simulink model "SingleStreamSSRwithPL"  (R2021a)
settings: Solver=VariableStepAuto  StartTime=0.0  StopTime=inf  RelTol=1e-3
PreLoadFcn:
  | xmcCheckSlxPath(bdroot)
  | SSR4_init
InitFcn:
  | xmcCheckSlxPath(bdroot)
  | SSR4_init;
undefined symbols (not defined in the file): c, FIR_MultiKernel_cin, FIR_MultiKernel_cincout, FIR_MultiKernel_cout, FramesPerVector, S, SHIFT_ACC, SingleStream, T, Taps, ValidDelay, VectorSize, vsva2197, xcvc1902
libraries: hdlBasic x84, aieBasic x28, simulink x25, aieUtilities x12, dspsrcs4 x1, vmcUtilities x1
(part 1 of 3)
settings Model: Creator=oliviert  LastModifiedBy=abehbood
settings SolverCC: AlgebraicLoopSolver=TrustRegion
settings DebuggingCC: SFMachineParentedDataDiag=warning

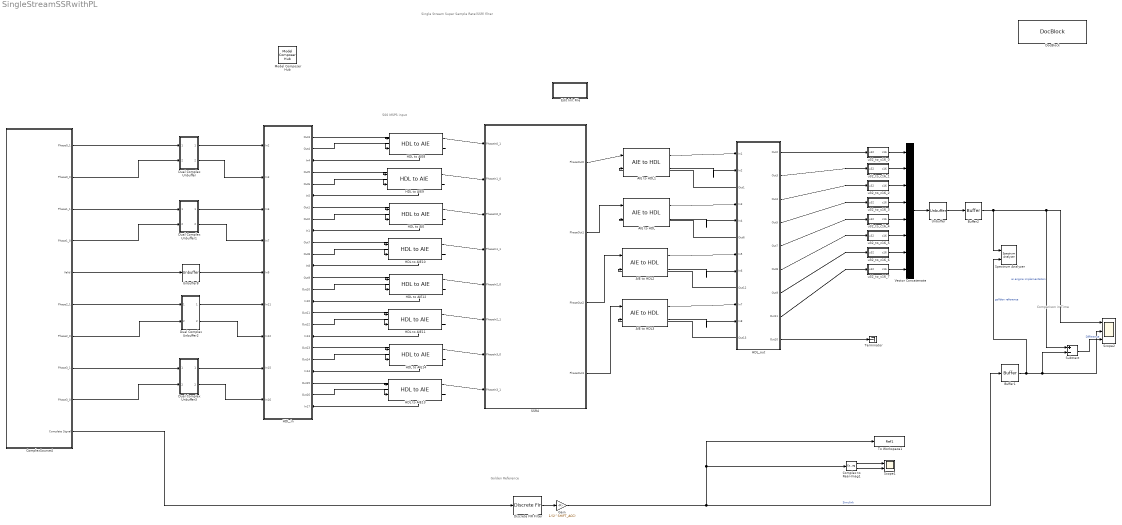
== system SingleStreamSSRwithPL ==
  note: Golden Reference
  note: Single Stream Super Sample Rate(SSR) filter
  note: Comparison in Time
  note: 500 MSPS input
  AIE to HDL{,1..3} (4 alike) : aieUtilities/AIE to HDL  OutDataType=uint64  OutSampleTime=1
  Buffer1 : Buffer  N=16  OutputFrames=off
  Buffer2 : Buffer  N=16  OutputFrames=off
  Complex to Real-Imag1 : ComplexToRealImag
  ComplexSource4 : Subsystem  mask{s=0}
      mask prompts: s "Seed"
  Discrete FIR Filter : DiscreteFir  Coefficients=Taps  InputProcessing=Columns as channels (frame based)
  DocBlock : simulink/Model-Wide Utilities/DocBlock  DocumentType=Text  mask(DocBlock){}
      content=|
      | ///////////////////////////////////////////////////////////////////////////
      | // Copyright 2020 Xilinx
      | //
      | // Licensed under the Apache License, Version 2.0 (the "License");
      | // you may not use this file except in compliance with the License.
      | // You may obtain a copy of the License at
      | //
      | // http://www.apache.org/licenses/LICENSE-2.0
      | //
      | // Unless required by applicable law or agreed to in writing, software
      | // distributed under the License is distributed on an "AS IS" BASIS,
      | // WITHOUT WARRANTIES OR CONDITIONS OF ANY KIND, either express or implied.
      | // See the License for the specific language governing permissions and
      | // limitations under the License.
      | ///////////////////////////////////////////////////////////////////////////
      mask Display:
      | xmcDrawBlockIcon();
      | disp(['{\fontsize{10pt}(c) Copyright 2020' ' Xilinx, Inc.}\newline \newline '],'texmode','on');
      | disp('{\fontsize{10pt}Licensed under the Apache License 2.0}','texmode','on');
      | disp('\newline \newline \newline{\fontsize{10pt}Double Click for Copyright Notice}','texmode','on');
  Dual Complex Unbuffer : Subsystem
  Dual Complex Unbuffer1 : Subsystem
  Dual Complex Unbuffer2 : Subsystem
  Dual Complex Unbuffer3 : Subsystem
  Edit Init File : Subsystem
      settings: OpenFcn=edit('SSR4_init.m');
  Gain : Gain  Gain=1/(2^SHIFT_ACC)
  HDL to AIE{,8..14} (8 alike) : aieUtilities/HDL to AIE  OutDataType=int16 (c)  OutSampleTime=4/T  SamplesPerFrame=4
  HDL_in : Subsystem
      settings: PortSchema="{\"entries\":[{\"content\":{\"sides\":[{\"content\":{\"connectorIds\":[\"In1\",\"In2\",\"In3\",\"In4\",\"In5\",\"In6\",\"In7\",\"In8\",\"In9\"]},\"type\":\"ConnectorPlacement.EquallySpacedRectSide\",\"uuid\":\"43963710-6fd6-4ca2-aef5-f578b9dcb653\"},{\"content\":{\"connectorIds\":[\"Out1\",\"Out2\",\"In10\",\"Out3\",\"Out4\",\"In11\",\"Out5\",\"Out6\",\"In12\",\"Out7\",\"Out8\",\"In13\",\"Out9\",\"Out10\",\"In14\",\"Out11\",\"Out12\",\"In15\",\"Out13\",\"Out14\",\"In16\",\"Out15\",\"Out16\",\"In17\"],\"side\":\"RIGHT\"},\"type\":\"ConnectorPlacement.EquallySpacedRectSide\",\"uuid\":\"a4fb1d0d-700c-40f1-8501-f280c21d0c52\"},{\"content\":{\"connectorIds\":[],\"side\":\"TOP\"},\"type\":\"ConnectorPlacement.EquallySpacedRectSide\",\"uuid\":\"ff581830-d8dd-44d7-ae40-7c0c1ac080ec\"}]},\"type\":\"ConnectorPlacement.EquallySpacedConnector\",\"uuid\":\"e2183898-06e4-482e-ae06-3d392b216275\"}],\"packageUris\":[\"http://schema.mathworks.com/mf0/Connector/R2020b\"],\"version\":\"1.0\"}"
  HDL_out : Subsystem
      settings: PortSchema="{\"entries\":[{\"content\":{\"sides\":[{\"content\":{\"connectorIds\":[\"In1\",\"In2\",\"Out10\",\"In3\",\"In4\",\"Out11\",\"In5\",\"In6\",\"Out12\",\"In7\",\"In8\",\"Out13\"]},\"type\":\"ConnectorPlacement.EquallySpacedRectSide\",\"uuid\":\"7f2474ee-a2a5-4d74-ae03-57eff4eca528\"},{\"content\":{\"connectorIds\":[\"Out1\",\"Out2\",\"Out3\",\"Out4\",\"Out5\",\"Out6\",\"Out7\",\"Out8\",\"Out9\"],\"side\":\"RIGHT\"},\"type\":\"ConnectorPlacement.EquallySpacedRectSide\",\"uuid\":\"05904fba-80d7-4be6-91c3-65cee4e3c770\"},{\"content\":{\"connectorIds\":[],\"side\":\"TOP\"},\"type\":\"ConnectorPlacement.EquallySpacedRectSide\",\"uuid\":\"ee8e52c5-3092-4f59-816b-8523dabda97a\"}]},\"type\":\"ConnectorPlacement.EquallySpacedConnector\",\"uuid\":\"7b2a5572-57fc-4b8c-a1f0-10ceb4480a97\"}],\"packageUris\":[\"http://schema.mathworks.com/mf0/Connector/R2020b\"],\"version\":\"1.0\"}"
  Model Composer Hub : vmcUtilities/Model Composer Hub  Tag=genX  CodeGeneration=off  SubsystemName=SSR4  TargetDirectory=./code  ExportType=AI Engines  IpVendor=xilinx.com  IpLibrary=hls  IpVersion=1.0  IpHWLanguage=Verilog  AieCompilerOptions={}  CreateTestbench=off  TestbenchStackSize=10  RunAieSim=off  AieSimTimeout=50000  RunAieSimProfiling=off  LaunchVitisAnalyzer=off  PlotOutput=off  RunX86Sim=off  X86SimTimeout=10  GenHwImage=off  PlatformType=Specify Platform  Platform=/proj/xbuilds/SWIP/2022.1_0310_2135/installs/lin64/Vitis/2022.1/base_platforms/xilinx_vck190_base_202210_1/xilinx_vck190_base_202210_1.xpfm  HwSystemType=Baremetal  HwValidationTarget=hw  ProjDevice=Versal VCK190 Evaluation Platform (xcvc1902-vsva2197-2MP-e-S)  ProjDevicePart=xcvc1902-vsva2197-2MP-e-S  SamplePeriod=-1  ClockFrequency=200  DataPathParallelism=1  xilinxfamily=versalaicore  part=xcvc1902  speed=-2MP-e-S  package=vsva2197  directory=./netlist  testbench=off  incr_netlist=off  synthesis_tool=Vivado  clock_wrapper=Clock Enables  dbl_ovrd=According to Block Masks  dcm_input_clock_period=10  sysclk_period=10  simulink_period=1  eval_field=0
  SSR4 : Subsystem
  Scope1 : Scope  NumInputPorts=2
  Scope2 : Scope  NumInputPorts=3
  Spectrum Analyzer : SpectrumAnalyzer  NumInputPorts=2
  Subtract : Sum  Inputs=+-
  Terminator : Terminator
  To Workspace1 : ToWorkspace  VariableName=Ref1  SampleTime=-1
      settings: Save2DSignal=2-D array (concatenate along first dimension)
  Unbuffer : Unbuffer
  Unbuffer8 : Unbuffer
  Vector Concatenate : Concatenate  NumInputs=8
  u32_to_c16_0 : Subsystem
  u32_to_c16_1 : Subsystem
  u32_to_c16_2 : Subsystem
  u32_to_c16_3 : Subsystem
  u32_to_c16_4 : Subsystem
  u32_to_c16_5 : Subsystem
  u32_to_c16_6 : Subsystem
  u32_to_c16_7 : Subsystem
  wires:
  ComplexSource4/10(Complete Signal) -> Discrete FIR Filter/1
  Discrete FIR Filter/1 -> Gain/1
  HDL to AIE/1 -> SSR4/3(PhaseIn0_0)
  HDL to AIE8/1 -> SSR4/1(PhaseIn0_1)
  HDL to AIE9/1 -> SSR4/2(PhaseIn1_0)
  HDL to AIE10/1 -> SSR4/4(PhaseIn1_1)
  HDL to AIE12/1 -> SSR4/5(PhaseIn2_0)
  HDL to AIE11/1 -> SSR4/6(PhaseIn2_1)
  HDL to AIE14/1 -> SSR4/7(PhaseIn3_0)
  HDL to AIE13/1 -> SSR4/8(PhaseIn3_1)
  Subtract/1 -> Scope2/3  "Difference"
  Complex to Real-Imag1/2 -> Scope1/2
  Complex to Real-Imag1/1 -> Scope1/1
  Gain/1 -> To Workspace1/1, Complex to Real-Imag1/1, Buffer1/1  "Simulink"
  Buffer1/1 -> Subtract/2, Scope2/2, Spectrum Analyzer/2  "gollden reference"
  Unbuffer/1 -> Buffer2/1
  Buffer2/1 -> Subtract/1, Scope2/1, Spectrum Analyzer/1  "ai engine implementation"
  ComplexSource4/1(Phase0_1) -> Dual Complex Unbuffer/1(P0_1)
  ComplexSource4/9(Phase3_0) -> Dual Complex Unbuffer3/2(P0_0)
  ComplexSource4/8(Phase3_1) -> Dual Complex Unbuffer3/1(P0_1)
  ComplexSource4/7(Phase2_0) -> Dual Complex Unbuffer2/2(P0_0)
  ComplexSource4/6(Phase2_1) -> Dual Complex Unbuffer2/1(P0_1)
  ComplexSource4/4(Phase1_0) -> Dual Complex Unbuffer1/2(P0_0)
  ComplexSource4/3(Phase1_1) -> Dual Complex Unbuffer1/1(P0_1)
  ComplexSource4/5(Valid) -> Unbuffer8/1
  ComplexSource4/2(Phase0_0) -> Dual Complex Unbuffer/2(P0_0)
  HDL to AIE/2 -> HDL_in/12(In1)
  Dual Complex Unbuffer/1(Out1) -> HDL_in/1(In2)
  Dual Complex Unbuffer/2(Out2) -> HDL_in/2(In3)
  HDL to AIE8/2 -> HDL_in/10(In4)
  HDL to AIE9/2 -> HDL_in/11(In5)
  Dual Complex Unbuffer1/1(Out1) -> HDL_in/3(In6)
  Dual Complex Unbuffer1/2(Out2) -> HDL_in/4(In7)
  HDL to AIE10/2 -> HDL_in/13(In8)
  Unbuffer8/1 -> HDL_in/5(In9)
  HDL to AIE12/2 -> HDL_in/14(In10)
  Dual Complex Unbuffer2/1(Out1) -> HDL_in/6(In11)
  Dual Complex Unbuffer2/2(Out2) -> HDL_in/7(In12)
  HDL to AIE11/2 -> HDL_in/15(In13)
  HDL to AIE14/2 -> HDL_in/16(In14)
  Dual Complex Unbuffer3/1(Out1) -> HDL_in/8(In15)
  Dual Complex Unbuffer3/2(Out2) -> HDL_in/9(In16)
  HDL to AIE13/2 -> HDL_in/17(In17)
  HDL_in/5(Out1) -> HDL to AIE/1
  HDL_in/6(Out2) -> HDL to AIE/2
  HDL_in/1(Out3) -> HDL to AIE8/1
  HDL_in/2(Out4) -> HDL to AIE8/2
  HDL_in/3(Out5) -> HDL to AIE9/1
  HDL_in/4(Out6) -> HDL to AIE9/2
  HDL_in/7(Out7) -> HDL to AIE10/1
  HDL_in/8(Out8) -> HDL to AIE10/2
  HDL_in/9(Out9) -> HDL to AIE12/1
  HDL_in/10(Out10) -> HDL to AIE12/2
  HDL_in/11(Out11) -> HDL to AIE11/1
  HDL_in/12(Out12) -> HDL to AIE11/2
  HDL_in/13(Out13) -> HDL to AIE14/1
  HDL_in/14(Out14) -> HDL to AIE14/2
  HDL_in/15(Out15) -> HDL to AIE13/1
  HDL_in/16(Out16) -> HDL to AIE13/2
  u32_to_c16_7/1(c16) -> Vector Concatenate/8
  u32_to_c16_6/1(c16) -> Vector Concatenate/7
  u32_to_c16_5/1(c16) -> Vector Concatenate/6
  u32_to_c16_4/1(c16) -> Vector Concatenate/5
  u32_to_c16_3/1(c16) -> Vector Concatenate/4
  u32_to_c16_2/1(c16) -> Vector Concatenate/3
  u32_to_c16_1/1(c16) -> Vector Concatenate/2
  u32_to_c16_0/1(c16) -> Vector Concatenate/1
  Vector Concatenate/1 -> Unbuffer/1
  SSR4/4(PhaseOut3) -> AIE to HDL3/1
  SSR4/3(PhaseOut2) -> AIE to HDL2/1
  SSR4/2(PhaseOut1) -> AIE to HDL/1
  SSR4/1(PhaseOut0) -> AIE to HDL1/1
  AIE to HDL1/1 -> HDL_out/1(In1)
  AIE to HDL1/2 -> HDL_out/2(In2)
  AIE to HDL/1 -> HDL_out/3(In3)
  AIE to HDL/2 -> HDL_out/4(In4)
  AIE to HDL2/1 -> HDL_out/5(In5)
  AIE to HDL2/2 -> HDL_out/6(In6)
  AIE to HDL3/1 -> HDL_out/7(In7)
  AIE to HDL3/2 -> HDL_out/8(In8)
  HDL_out/10(Out1) -> AIE to HDL1/2
  HDL_out/1(Out2) -> u32_to_c16_0/1(u32)
  HDL_out/2(Out3) -> u32_to_c16_1/1(u32)
  HDL_out/3(Out4) -> u32_to_c16_2/1(u32)
  HDL_out/4(Out5) -> u32_to_c16_3/1(u32)
  HDL_out/11(Out6) -> AIE to HDL/2
  HDL_out/5(Out7) -> u32_to_c16_4/1(u32)
  HDL_out/6(Out8) -> u32_to_c16_5/1(u32)
  HDL_out/7(Out9) -> u32_to_c16_6/1(u32)
  HDL_out/9(Out10) -> Terminator/1
  HDL_out/8(Out11) -> u32_to_c16_7/1(u32)
  HDL_out/12(Out12) -> AIE to HDL2/2
  HDL_out/13(Out13) -> AIE to HDL3/2

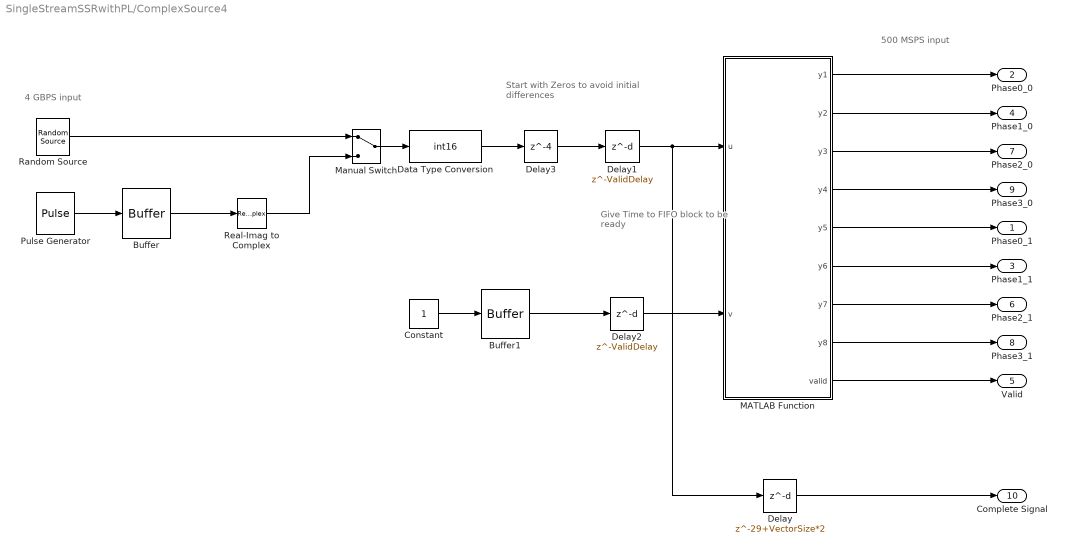
== system SingleStreamSSRwithPL/ComplexSource4 ==
  note: Give Time to
      | FIFO block
      | to be ready
  note: Start with Zeros
      | to avoid
      | initial differences
  note: 4 GBPS input
  note: 500 MSPS input
  Buffer : Buffer  N=VectorSize  OutputFrames=off
  Buffer1 : Buffer  N=FramesPerVector  OutputFrames=off
  Constant : Constant  SampleTime=1
  Data Type Conversion : DataTypeConversion  OutDataTypeStr=int16
  Delay : Delay  DelayLength=29+VectorSize*2  InputProcessing=Columns as channels (frame based)
  Delay1 : Delay  DelayLength=ValidDelay
  Delay2 : Delay  DelayLength=ValidDelay
  Delay3 : Delay  DelayLength=4
  MATLAB Function : MATLAB Function  TreatAsAtomicUnit=on
  Manual Switch : ManualSwitch
  Pulse Generator : DiscretePulseGenerator  Amplitude=20000  Period=32 + 40*5  PhaseDelay=32  SampleTime=1/T
  Random Source : dspsrcs4/Random Source  SrcType=Uniform  NormMethod=Ziggurat  CltLength=12  MinVal=-20000  MaxVal=20000  MeanVal=0  VarVal=1  RepMode=Specify seed  rawSeed=s  IsInherit=off  SampMode=Discrete  SampTime=1/T  SampFrame=VectorSize  DataType=Double  OutComplex=Complex  OutputFrames=off
  Real-Imag to Complex : RealImagToComplex  Input=Real
  Phase0_1 : Outport
  Phase0_0 : Outport  Port=2
  Phase1_1 : Outport  Port=3
  Phase1_0 : Outport  Port=4
  Valid : Outport  Port=5
  Phase2_1 : Outport  Port=6
  Phase2_0 : Outport  Port=7
  Phase3_1 : Outport  Port=8
  Phase3_0 : Outport  Port=9
  Complete Signal : Outport  Port=10
  wires:
  MATLAB Function/1(y1) -> Phase0_0/1
  MATLAB Function/2(y2) -> Phase1_0/1
  MATLAB Function/3(y3) -> Phase2_0/1
  MATLAB Function/4(y4) -> Phase3_0/1
  Real-Imag to Complex/1 -> Manual Switch/2
  Pulse Generator/1 -> Buffer/1
  Delay/1 -> Complete Signal/1
  Buffer/1 -> Real-Imag to Complex/1
  Manual Switch/1 -> Data Type Conversion/1
  MATLAB Function/9(valid) -> Valid/1
  MATLAB Function/8(y8) -> Phase3_1/1
  MATLAB Function/7(y7) -> Phase2_1/1
  MATLAB Function/6(y6) -> Phase1_1/1
  MATLAB Function/5(y5) -> Phase0_1/1
  Random Source/1 -> Manual Switch/1
  Delay1/1 -> Delay/1, MATLAB Function/1(u)
  Delay2/1 -> MATLAB Function/2(v)
  Constant/1 -> Buffer1/1
  Buffer1/1 -> Delay2/1
  Data Type Conversion/1 -> Delay3/1
  Delay3/1 -> Delay1/1

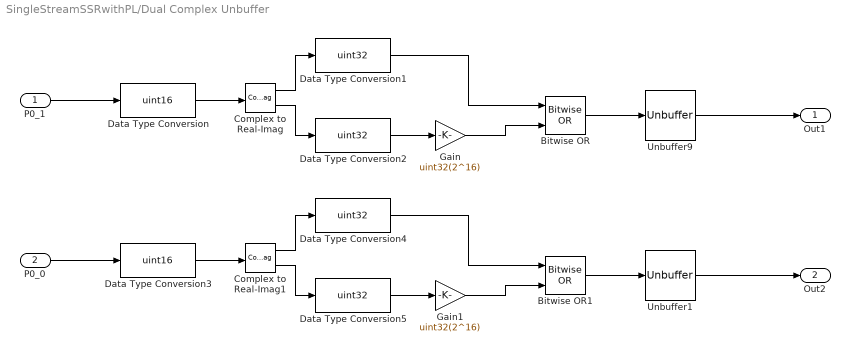
== system SingleStreamSSRwithPL/Dual Complex Unbuffer ==
  P0_1 : Inport
  P0_0 : Inport  Port=2
  Bitwise OR : simulink/Logic and Bit Operations/Bitwise Operator  logicop=OR  UseBitMask=off  NumInputPorts=2  BitMask=bin2dec('11011001')  BitMaskRealWorld=Stored Integer
  Bitwise OR1 : simulink/Logic and Bit Operations/Bitwise Operator  logicop=OR  UseBitMask=off  NumInputPorts=2  BitMask=bin2dec('11011001')  BitMaskRealWorld=Stored Integer
  Complex to Real-Imag : ComplexToRealImag
  Complex to Real-Imag1 : ComplexToRealImag
  Data Type Conversion : DataTypeConversion  OutDataTypeStr=uint16  ConvertRealWorld=Stored Integer (SI)
  Data Type Conversion{1..2,4..5} (4 alike) : DataTypeConversion  OutDataTypeStr=uint32  ConvertRealWorld=Stored Integer (SI)
  Data Type Conversion3 : DataTypeConversion  OutDataTypeStr=uint16  ConvertRealWorld=Stored Integer (SI)
  Gain : Gain  Gain=uint32(2^16)  OutDataTypeStr=uint32
  Gain1 : Gain  Gain=uint32(2^16)  OutDataTypeStr=uint32
  Unbuffer1 : Unbuffer
  Unbuffer9 : Unbuffer
  Out1 : Outport
  Out2 : Outport  Port=2
  wires:
  Unbuffer1/1 -> Out2/1
  Unbuffer9/1 -> Out1/1
  Data Type Conversion/1 -> Complex to Real-Imag/1
  P0_1/1 -> Data Type Conversion/1
  Data Type Conversion2/1 -> Gain/1
  Bitwise OR/1 -> Unbuffer9/1
  Complex to Real-Imag/1 -> Data Type Conversion1/1
  Complex to Real-Imag/2 -> Data Type Conversion2/1
  Data Type Conversion1/1 -> Bitwise OR/1
  Gain/1 -> Bitwise OR/2
  Gain1/1 -> Bitwise OR1/2
  Data Type Conversion4/1 -> Bitwise OR1/1
  Complex to Real-Imag1/2 -> Data Type Conversion5/1
  Complex to Real-Imag1/1 -> Data Type Conversion4/1
  Data Type Conversion5/1 -> Gain1/1
  Data Type Conversion3/1 -> Complex to Real-Imag1/1
  P0_0/1 -> Data Type Conversion3/1
  Bitwise OR1/1 -> Unbuffer1/1

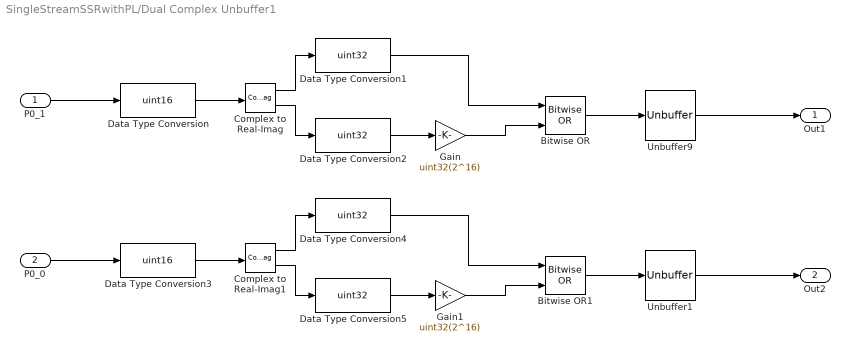
== system SingleStreamSSRwithPL/Dual Complex Unbuffer1 ==
  P0_1 : Inport
  P0_0 : Inport  Port=2
  Bitwise OR : simulink/Logic and Bit Operations/Bitwise Operator  logicop=OR  UseBitMask=off  NumInputPorts=2  BitMask=bin2dec('11011001')  BitMaskRealWorld=Stored Integer
  Bitwise OR1 : simulink/Logic and Bit Operations/Bitwise Operator  logicop=OR  UseBitMask=off  NumInputPorts=2  BitMask=bin2dec('11011001')  BitMaskRealWorld=Stored Integer
  Complex to Real-Imag : ComplexToRealImag
  Complex to Real-Imag1 : ComplexToRealImag
  Data Type Conversion : DataTypeConversion  OutDataTypeStr=uint16  ConvertRealWorld=Stored Integer (SI)
  Data Type Conversion{1..2,4..5} (4 alike) : DataTypeConversion  OutDataTypeStr=uint32  ConvertRealWorld=Stored Integer (SI)
  Data Type Conversion3 : DataTypeConversion  OutDataTypeStr=uint16  ConvertRealWorld=Stored Integer (SI)
  Gain : Gain  Gain=uint32(2^16)  OutDataTypeStr=uint32
  Gain1 : Gain  Gain=uint32(2^16)  OutDataTypeStr=uint32
  Unbuffer1 : Unbuffer
  Unbuffer9 : Unbuffer
  Out1 : Outport
  Out2 : Outport  Port=2
  wires:
  Bitwise OR1/1 -> Unbuffer1/1
  P0_0/1 -> Data Type Conversion3/1
  Data Type Conversion3/1 -> Complex to Real-Imag1/1
  Data Type Conversion5/1 -> Gain1/1
  Complex to Real-Imag1/1 -> Data Type Conversion4/1
  Complex to Real-Imag1/2 -> Data Type Conversion5/1
  Data Type Conversion4/1 -> Bitwise OR1/1
  Gain1/1 -> Bitwise OR1/2
  Gain/1 -> Bitwise OR/2
  Data Type Conversion1/1 -> Bitwise OR/1
  Complex to Real-Imag/2 -> Data Type Conversion2/1
  Complex to Real-Imag/1 -> Data Type Conversion1/1
  Bitwise OR/1 -> Unbuffer9/1
  Data Type Conversion2/1 -> Gain/1
  P0_1/1 -> Data Type Conversion/1
  Data Type Conversion/1 -> Complex to Real-Imag/1
  Unbuffer9/1 -> Out1/1
  Unbuffer1/1 -> Out2/1

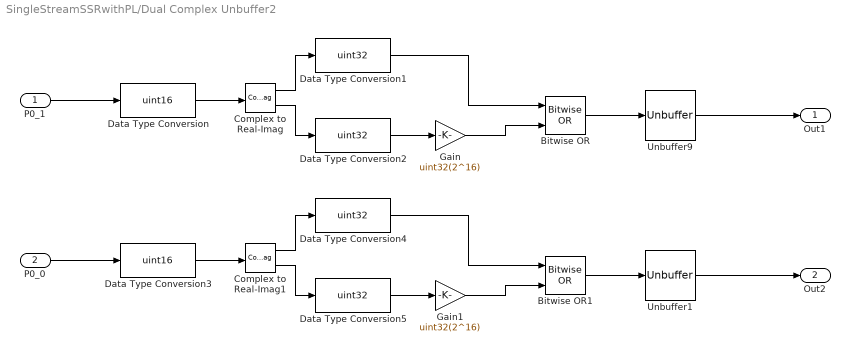
== system SingleStreamSSRwithPL/Dual Complex Unbuffer2 ==
  P0_1 : Inport
  P0_0 : Inport  Port=2
  Bitwise OR : simulink/Logic and Bit Operations/Bitwise Operator  logicop=OR  UseBitMask=off  NumInputPorts=2  BitMask=bin2dec('11011001')  BitMaskRealWorld=Stored Integer
  Bitwise OR1 : simulink/Logic and Bit Operations/Bitwise Operator  logicop=OR  UseBitMask=off  NumInputPorts=2  BitMask=bin2dec('11011001')  BitMaskRealWorld=Stored Integer
  Complex to Real-Imag : ComplexToRealImag
  Complex to Real-Imag1 : ComplexToRealImag
  Data Type Conversion : DataTypeConversion  OutDataTypeStr=uint16  ConvertRealWorld=Stored Integer (SI)
  Data Type Conversion{1..2,4..5} (4 alike) : DataTypeConversion  OutDataTypeStr=uint32  ConvertRealWorld=Stored Integer (SI)
  Data Type Conversion3 : DataTypeConversion  OutDataTypeStr=uint16  ConvertRealWorld=Stored Integer (SI)
  Gain : Gain  Gain=uint32(2^16)  OutDataTypeStr=uint32
  Gain1 : Gain  Gain=uint32(2^16)  OutDataTypeStr=uint32
  Unbuffer1 : Unbuffer
  Unbuffer9 : Unbuffer
  Out1 : Outport
  Out2 : Outport  Port=2
  wires:
  Bitwise OR1/1 -> Unbuffer1/1
  P0_0/1 -> Data Type Conversion3/1
  Data Type Conversion3/1 -> Complex to Real-Imag1/1
  Data Type Conversion5/1 -> Gain1/1
  Complex to Real-Imag1/1 -> Data Type Conversion4/1
  Complex to Real-Imag1/2 -> Data Type Conversion5/1
  Data Type Conversion4/1 -> Bitwise OR1/1
  Gain1/1 -> Bitwise OR1/2
  Gain/1 -> Bitwise OR/2
  Data Type Conversion1/1 -> Bitwise OR/1
  Complex to Real-Imag/2 -> Data Type Conversion2/1
  Complex to Real-Imag/1 -> Data Type Conversion1/1
  Bitwise OR/1 -> Unbuffer9/1
  Data Type Conversion2/1 -> Gain/1
  P0_1/1 -> Data Type Conversion/1
  Data Type Conversion/1 -> Complex to Real-Imag/1
  Unbuffer9/1 -> Out1/1
  Unbuffer1/1 -> Out2/1

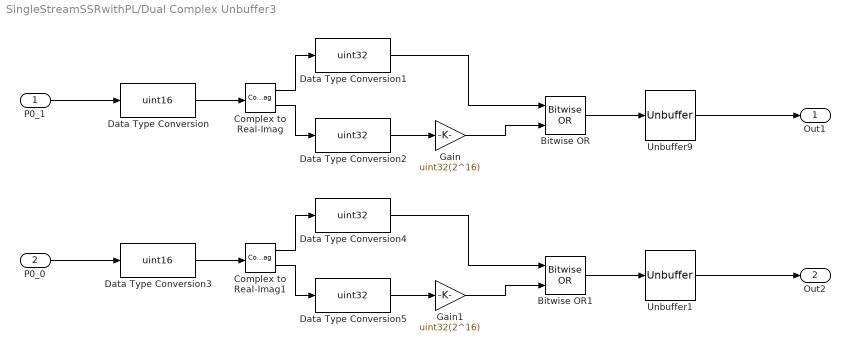
== system SingleStreamSSRwithPL/Dual Complex Unbuffer3 ==
  P0_1 : Inport
  P0_0 : Inport  Port=2
  Bitwise OR : simulink/Logic and Bit Operations/Bitwise Operator  logicop=OR  UseBitMask=off  NumInputPorts=2  BitMask=bin2dec('11011001')  BitMaskRealWorld=Stored Integer
  Bitwise OR1 : simulink/Logic and Bit Operations/Bitwise Operator  logicop=OR  UseBitMask=off  NumInputPorts=2  BitMask=bin2dec('11011001')  BitMaskRealWorld=Stored Integer
  Complex to Real-Imag : ComplexToRealImag
  Complex to Real-Imag1 : ComplexToRealImag
  Data Type Conversion : DataTypeConversion  OutDataTypeStr=uint16  ConvertRealWorld=Stored Integer (SI)
  Data Type Conversion{1..2,4..5} (4 alike) : DataTypeConversion  OutDataTypeStr=uint32  ConvertRealWorld=Stored Integer (SI)
  Data Type Conversion3 : DataTypeConversion  OutDataTypeStr=uint16  ConvertRealWorld=Stored Integer (SI)
  Gain : Gain  Gain=uint32(2^16)  OutDataTypeStr=uint32
  Gain1 : Gain  Gain=uint32(2^16)  OutDataTypeStr=uint32
  Unbuffer1 : Unbuffer
  Unbuffer9 : Unbuffer
  Out1 : Outport
  Out2 : Outport  Port=2
  wires:
  Bitwise OR1/1 -> Unbuffer1/1
  P0_0/1 -> Data Type Conversion3/1
  Data Type Conversion3/1 -> Complex to Real-Imag1/1
  Data Type Conversion5/1 -> Gain1/1
  Complex to Real-Imag1/1 -> Data Type Conversion4/1
  Complex to Real-Imag1/2 -> Data Type Conversion5/1
  Data Type Conversion4/1 -> Bitwise OR1/1
  Gain1/1 -> Bitwise OR1/2
  Gain/1 -> Bitwise OR/2
  Data Type Conversion1/1 -> Bitwise OR/1
  Complex to Real-Imag/2 -> Data Type Conversion2/1
  Complex to Real-Imag/1 -> Data Type Conversion1/1
  Bitwise OR/1 -> Unbuffer9/1
  Data Type Conversion2/1 -> Gain/1
  P0_1/1 -> Data Type Conversion/1
  Data Type Conversion/1 -> Complex to Real-Imag/1
  Unbuffer9/1 -> Out1/1
  Unbuffer1/1 -> Out2/1

== system SingleStreamSSRwithPL/Edit Init File ==

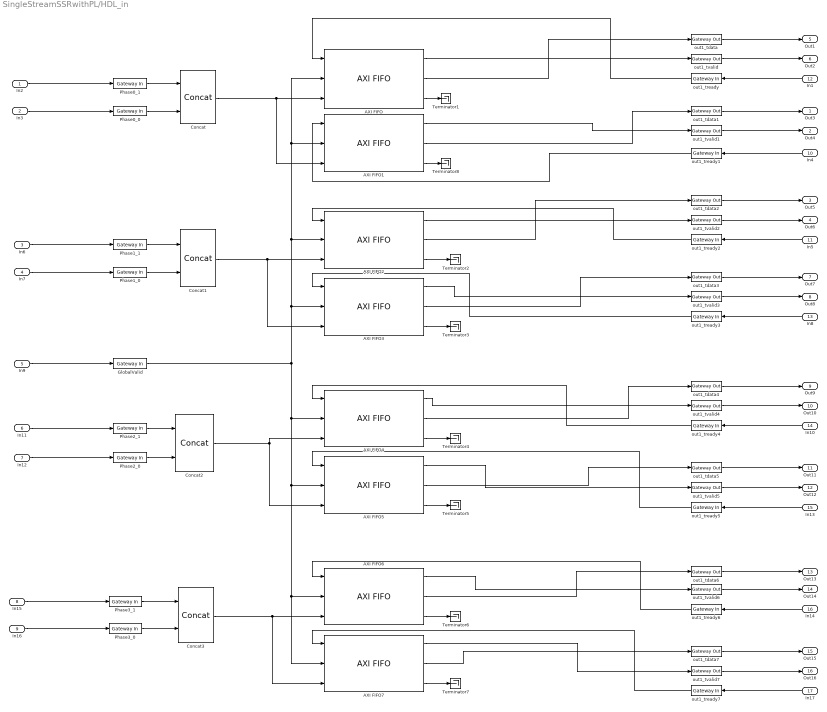
== system SingleStreamSSRwithPL/HDL_in ==
  In2 : Inport
  In3 : Inport  Port=2
  In6 : Inport  Port=3
  In7 : Inport  Port=4
  In9 : Inport  Port=5
  In11 : Inport  Port=6
  In12 : Inport  Port=7
  In15 : Inport  Port=8
  In16 : Inport  Port=9
  In4 : Inport  Port=10
  In5 : Inport  Port=11
  In1 : Inport  Port=12
  In8 : Inport  Port=13
  In10 : Inport  Port=14
  In13 : Inport  Port=15
  In14 : Inport  Port=16
  In17 : Inport  Port=17
  AXI FIFO{,1..7} (8 alike) : hdlBasic/AXI FIFO  input_depth_axis=512  actual_fifo_depth_label=514  enable_tdata=on  enable_tdest=off  enable_tstrb=off  enable_tready=on  enable_tid=off  enable_tuser=off  enable_tkeep=off  enable_tlast=off  has_aresetn=off  enable_data_counts_axis=off  fifo_implementation_type_axis=Common Clock Block RAM  trim_axipin_name=on  programmable_full_type_axis=Full  full_threshold_assert_value_axis=0  programmable_empty_type_axis=Empty  empty_threshold_assert_value_axis=1022  underflow_flag_axi=0  underflow_sense_axi=Active High  overflow_flag_axi=0  overflow_sense_axi=Active High  simulation_type=fast_sim  XmcBlockStatus=1  maskContainerNames=tabcontainer1  block_type=axi_fifo  block_config=sysgen:AXI_FIFO_config
  Concat{,1..3} (4 alike) : hdlBasic/Concat  num_inputs=2  XmcBlockStatus=1  maskContainerNames=group1  block_type=concat  block_config=sysgen:Concat_config
  GlobalValid : hdlBasic/Gateway In  gui_display_data_type=Boolean  arith_type=Boolean  n_bits=16  bin_pt=14  preci_type=Single  exp_width=8  frac_width=24  rows=1  columns=1  quantization="Round  (unbiased: +/- Inf)"  overflow=Saturate  period=1  UseAsADC=off  ADCChannel='1'  interface=None  automatic_assignment=on  address_offset=hex2dec('00')  intf_name=''  intf_description=''  default_value=0  timing_constraint=None  locs_specified=off  LOCs={}  io_standard={}  inherit_from_input=off  hdl_port=on  XmcBlockStatus=1  maskContainerNames=group4  block_type=gatewayin  block_config=sysgen:gateway_in_config
  Phase0_0 : hdlBasic/Gateway In  gui_display_data_type=Fixed-point  arith_type=Unsigned  n_bits=32  bin_pt=0  preci_type=Single  exp_width=8  frac_width=24  rows=1  columns=1  quantization="Round  (unbiased: +/- Inf)"  overflow=Saturate  period=1  UseAsADC=off  ADCChannel='1'  interface=None  automatic_assignment=on  address_offset=hex2dec('00')  intf_name=''  intf_description=''  default_value=0  timing_constraint=None  locs_specified=off  LOCs={}  io_standard={}  inherit_from_input=off  hdl_port=on  XmcBlockStatus=1  maskContainerNames=group4  block_type=gatewayin  block_config=sysgen:gateway_in_config
  Phase0_1 : hdlBasic/Gateway In  gui_display_data_type=Fixed-point  arith_type=Unsigned  n_bits=32  bin_pt=0  preci_type=Single  exp_width=8  frac_width=24  rows=1  columns=1  quantization="Round  (unbiased: +/- Inf)"  overflow=Saturate  period=1  UseAsADC=off  ADCChannel='1'  interface=None  automatic_assignment=on  address_offset=hex2dec('00')  intf_name=''  intf_description=''  default_value=0  timing_constraint=None  locs_specified=off  LOCs={}  io_standard={}  inherit_from_input=off  hdl_port=on  XmcBlockStatus=1  maskContainerNames=group4  block_type=gatewayin  block_config=sysgen:gateway_in_config
  Phase1_0 : hdlBasic/Gateway In  gui_display_data_type=Fixed-point  arith_type=Unsigned  n_bits=32  bin_pt=0  preci_type=Single  exp_width=8  frac_width=24  rows=1  columns=1  quantization="Round  (unbiased: +/- Inf)"  overflow=Saturate  period=1  UseAsADC=off  ADCChannel='1'  interface=None  automatic_assignment=on  address_offset=hex2dec('00')  intf_name=''  intf_description=''  default_value=0  timing_constraint=None  locs_specified=off  LOCs={}  io_standard={}  inherit_from_input=off  hdl_port=on  XmcBlockStatus=1  maskContainerNames=group4  block_type=gatewayin  block_config=sysgen:gateway_in_config
  Phase1_1 : hdlBasic/Gateway In  gui_display_data_type=Fixed-point  arith_type=Unsigned  n_bits=32  bin_pt=0  preci_type=Single  exp_width=8  frac_width=24  rows=1  columns=1  quantization="Round  (unbiased: +/- Inf)"  overflow=Saturate  period=1  UseAsADC=off  ADCChannel='1'  interface=None  automatic_assignment=on  address_offset=hex2dec('00')  intf_name=''  intf_description=''  default_value=0  timing_constraint=None  locs_specified=off  LOCs={}  io_standard={}  inherit_from_input=off  hdl_port=on  XmcBlockStatus=1  maskContainerNames=group4  block_type=gatewayin  block_config=sysgen:gateway_in_config
  Phase2_0 : hdlBasic/Gateway In  gui_display_data_type=Fixed-point  arith_type=Unsigned  n_bits=32  bin_pt=0  preci_type=Single  exp_width=8  frac_width=24  rows=1  columns=1  quantization="Round  (unbiased: +/- Inf)"  overflow=Saturate  period=1  UseAsADC=off  ADCChannel='1'  interface=None  automatic_assignment=on  address_offset=hex2dec('00')  intf_name=''  intf_description=''  default_value=0  timing_constraint=None  locs_specified=off  LOCs={}  io_standard={}  inherit_from_input=off  hdl_port=on  XmcBlockStatus=1  maskContainerNames=group4  block_type=gatewayin  block_config=sysgen:gateway_in_config
  Phase2_1 : hdlBasic/Gateway In  gui_display_data_type=Fixed-point  arith_type=Unsigned  n_bits=32  bin_pt=0  preci_type=Single  exp_width=8  frac_width=24  rows=1  columns=1  quantization="Round  (unbiased: +/- Inf)"  overflow=Saturate  period=1  UseAsADC=off  ADCChannel='1'  interface=None  automatic_assignment=on  address_offset=hex2dec('00')  intf_name=''  intf_description=''  default_value=0  timing_constraint=None  locs_specified=off  LOCs={}  io_standard={}  inherit_from_input=off  hdl_port=on  XmcBlockStatus=1  maskContainerNames=group4  block_type=gatewayin  block_config=sysgen:gateway_in_config
  Phase3_0 : hdlBasic/Gateway In  gui_display_data_type=Fixed-point  arith_type=Unsigned  n_bits=32  bin_pt=0  preci_type=Single  exp_width=8  frac_width=24  rows=1  columns=1  quantization="Round  (unbiased: +/- Inf)"  overflow=Saturate  period=1  UseAsADC=off  ADCChannel='1'  interface=None  automatic_assignment=on  address_offset=hex2dec('00')  intf_name=''  intf_description=''  default_value=0  timing_constraint=None  locs_specified=off  LOCs={}  io_standard={}  inherit_from_input=off  hdl_port=on  XmcBlockStatus=1  maskContainerNames=group4  block_type=gatewayin  block_config=sysgen:gateway_in_config
  Phase3_1 : hdlBasic/Gateway In  gui_display_data_type=Fixed-point  arith_type=Unsigned  n_bits=32  bin_pt=0  preci_type=Single  exp_width=8  frac_width=24  rows=1  columns=1  quantization="Round  (unbiased: +/- Inf)"  overflow=Saturate  period=1  UseAsADC=off  ADCChannel='1'  interface=None  automatic_assignment=on  address_offset=hex2dec('00')  intf_name=''  intf_description=''  default_value=0  timing_constraint=None  locs_specified=off  LOCs={}  io_standard={}  inherit_from_input=off  hdl_port=on  XmcBlockStatus=1  maskContainerNames=group4  block_type=gatewayin  block_config=sysgen:gateway_in_config
  Terminator{1..8} (8 alike) : Terminator
  out1_tdata{,1..7} (8 alike) : hdlBasic/Gateway Out  inherit_from_input=on  hdl_port=on  rows=1  columns=1  UseAsDAC=off  DACChannel='1'  interface=None  automatic_assignment=on  address_offset=hex2dec('00')  intf_name=''  intf_description=''  timing_constraint=None  locs_specified=off  LOCs={}  io_standard={}  XmcBlockStatus=1  maskContainerNames=group4  block_type=gatewayout  block_config=sysgen:gateway_out_config
  out1_tready{,1..7} (8 alike) : hdlBasic/Gateway In  gui_display_data_type=Boolean  arith_type=Boolean  n_bits=16  bin_pt=14  preci_type=Single  exp_width=8  frac_width=24  rows=1  columns=1  quantization="Round  (unbiased: +/- Inf)"  overflow=Saturate  period=1  UseAsADC=off  ADCChannel='1'  interface=None  automatic_assignment=on  address_offset=hex2dec('00')  intf_name=''  intf_description=''  default_value=0  timing_constraint=None  locs_specified=off  LOCs={}  io_standard={}  inherit_from_input=off  hdl_port=on  XmcBlockStatus=1  maskContainerNames=group4  block_type=gatewayin  block_config=sysgen:gateway_in_config
  out1_tvalid{,1..7} (8 alike) : hdlBasic/Gateway Out  inherit_from_input=on  hdl_port=on  rows=1  columns=1  UseAsDAC=off  DACChannel='1'  interface=None  automatic_assignment=on  address_offset=hex2dec('00')  intf_name=''  intf_description=''  timing_constraint=None  locs_specified=off  LOCs={}  io_standard={}  XmcBlockStatus=1  maskContainerNames=group4  block_type=gatewayout  block_config=sysgen:gateway_out_config
  Out3 : Outport
  Out4 : Outport  Port=2
  Out5 : Outport  Port=3
  Out6 : Outport  Port=4
  Out1 : Outport  Port=5
  Out2 : Outport  Port=6
  Out7 : Outport  Port=7
  Out8 : Outport  Port=8
  Out9 : Outport  Port=9
  Out10 : Outport  Port=10
  Out11 : Outport  Port=11
  Out12 : Outport  Port=12
  Out13 : Outport  Port=13
  Out14 : Outport  Port=14
  Out15 : Outport  Port=15
  Out16 : Outport  Port=16
  wires:
  out1_tdata3/1 -> Out7/1
  AXI FIFO5/1 -> out1_tvalid5/1
  In5/1 -> out1_tready2/1
  AXI FIFO4/3 -> Terminator4/1
  Phase3_0/1 -> Concat3/2
  out1_tready2/1 -> AXI FIFO2/1
  out1_tdata/1 -> Out1/1
  AXI FIFO6/1 -> out1_tvalid6/1
  In2/1 -> Phase0_1/1
  In16/1 -> Phase3_0/1
  In7/1 -> Phase1_0/1
  AXI FIFO1/3 -> Terminator8/1
  AXI FIFO5/2 -> out1_tdata5/1
  AXI FIFO6/3 -> Terminator6/1
  Phase0_1/1 -> Concat/1
  AXI FIFO4/2 -> out1_tdata4/1
  AXI FIFO/2 -> out1_tdata/1
  AXI FIFO4/1 -> out1_tvalid4/1
  out1_tdata5/1 -> Out11/1
  out1_tready6/1 -> AXI FIFO6/1
  out1_tready5/1 -> AXI FIFO5/1
  Phase3_1/1 -> Concat3/1
  out1_tvalid1/1 -> Out4/1
  AXI FIFO7/2 -> out1_tdata7/1
  out1_tdata6/1 -> Out13/1
  out1_tvalid7/1 -> Out16/1
  In12/1 -> Phase2_0/1
  out1_tready1/1 -> AXI FIFO1/1
  In15/1 -> Phase3_1/1
  out1_tvalid4/1 -> Out10/1
  AXI FIFO7/3 -> Terminator7/1
  In11/1 -> Phase2_1/1
  In4/1 -> out1_tready1/1
  AXI FIFO/3 -> Terminator1/1
  GlobalValid/1 -> AXI FIFO4/2, AXI FIFO6/2, AXI FIFO7/2, AXI FIFO5/2, AXI FIFO3/2, AXI FIFO2/2, AXI FIFO1/2, AXI FIFO/2
  AXI FIFO3/3 -> Terminator3/1
  out1_tready/1 -> AXI FIFO/1
  AXI FIFO3/1 -> out1_tvalid3/1
  out1_tdata1/1 -> Out3/1
  out1_tvalid3/1 -> Out8/1
  In13/1 -> out1_tready5/1
  Phase2_1/1 -> Concat2/1
  AXI FIFO2/1 -> out1_tvalid2/1
  In8/1 -> out1_tready3/1
  AXI FIFO/1 -> out1_tvalid/1
  In14/1 -> out1_tready6/1
  Phase1_1/1 -> Concat1/1
  In1/1 -> out1_tready/1
  out1_tvalid5/1 -> Out12/1
  In17/1 -> out1_tready7/1
  In10/1 -> out1_tready4/1
  Concat3/1 -> AXI FIFO7/3, AXI FIFO6/3
  AXI FIFO2/2 -> out1_tdata2/1
  out1_tready3/1 -> AXI FIFO3/1
  In6/1 -> Phase1_1/1
  In3/1 -> Phase0_0/1
  AXI FIFO7/1 -> out1_tvalid7/1
  In9/1 -> GlobalValid/1
  Concat2/1 -> AXI FIFO4/3, AXI FIFO5/3
  AXI FIFO2/3 -> Terminator2/1
  out1_tready7/1 -> AXI FIFO7/1
  out1_tdata4/1 -> Out9/1
  Concat/1 -> AXI FIFO1/3, AXI FIFO/3
  Concat1/1 -> AXI FIFO2/3, AXI FIFO3/3
  out1_tvalid2/1 -> Out6/1
  Phase2_0/1 -> Concat2/2
  AXI FIFO3/2 -> out1_tdata3/1
  Phase0_0/1 -> Concat/2
  AXI FIFO5/3 -> Terminator5/1
  AXI FIFO1/1 -> out1_tvalid1/1
  AXI FIFO6/2 -> out1_tdata6/1
  Phase1_0/1 -> Concat1/2
  out1_tdata7/1 -> Out15/1
  out1_tvalid6/1 -> Out14/1
  out1_tvalid/1 -> Out2/1
  out1_tdata2/1 -> Out5/1
  AXI FIFO1/2 -> out1_tdata1/1
  out1_tready4/1 -> AXI FIFO4/1

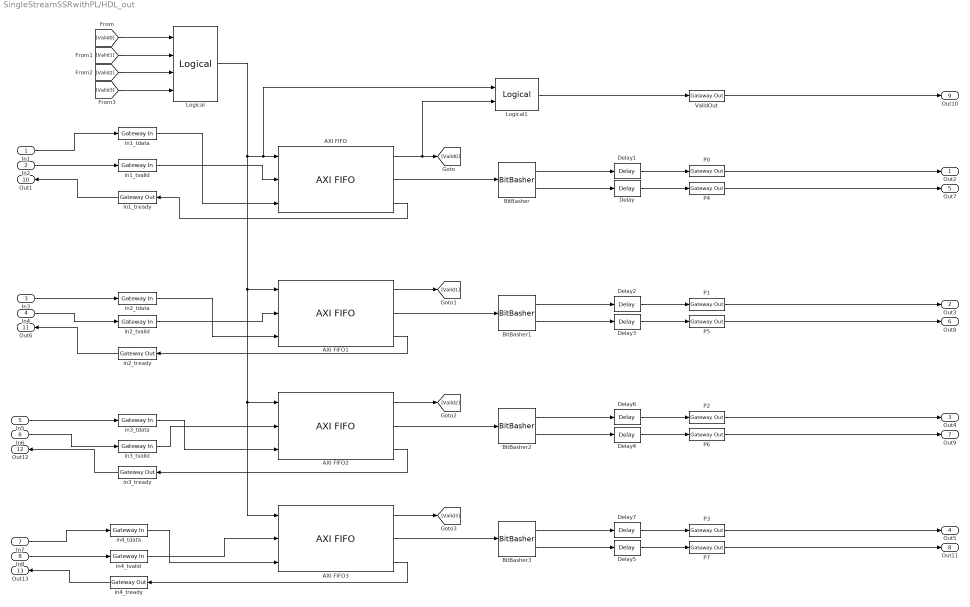
== system SingleStreamSSRwithPL/HDL_out ==
  In1 : Inport
  In2 : Inport  Port=2
  In3 : Inport  Port=3
  In4 : Inport  Port=4
  In5 : Inport  Port=5
  In6 : Inport  Port=6
  In7 : Inport  Port=7
  In8 : Inport  Port=8
  AXI FIFO{,1..3} (4 alike) : hdlBasic/AXI FIFO  input_depth_axis=512  actual_fifo_depth_label=514  enable_tdata=on  enable_tdest=off  enable_tstrb=off  enable_tready=on  enable_tid=off  enable_tuser=off  enable_tkeep=off  enable_tlast=off  has_aresetn=off  enable_data_counts_axis=off  fifo_implementation_type_axis=Common Clock Block RAM  trim_axipin_name=on  programmable_full_type_axis=Full  full_threshold_assert_value_axis=0  programmable_empty_type_axis=Empty  empty_threshold_assert_value_axis=1022  underflow_flag_axi=0  underflow_sense_axi=Active High  overflow_flag_axi=0  overflow_sense_axi=Active High  simulation_type=fast_sim  XmcBlockStatus=1  maskContainerNames=tabcontainer1  block_type=axi_fifo  block_config=sysgen:AXI_FIFO_config
  BitBasher : hdlBasic/BitBasher  bitexpr=|  display_expr=off  sr_1=lo  arith_type1=Unsigned  bin_pt1=0  sr_2=hi  arith_type2=Unsigned  bin_pt2=0  sr_3=3  arith_type3=Unsigned  bin_pt3=0  sr_4=4  arith_type4=Unsigned  bin_pt4=0  XmcBlockStatus=1  maskContainerNames=group1  block_type=bitbasher  block_config=sysgen:BitBasher_config
      | lo={in[31:0]}
      | hi={in[63:32]}
  BitBasher1 : hdlBasic/BitBasher  bitexpr=|  display_expr=off  sr_1=lo  arith_type1=Unsigned  bin_pt1=0  sr_2=hi  arith_type2=Unsigned  bin_pt2=0  sr_3=3  arith_type3=Unsigned  bin_pt3=0  sr_4=4  arith_type4=Unsigned  bin_pt4=0  XmcBlockStatus=1  maskContainerNames=group1  block_type=bitbasher  block_config=sysgen:BitBasher_config
      | lo={in[31:0]}
      | hi={in[63:32]}
  BitBasher2 : hdlBasic/BitBasher  bitexpr=|  display_expr=off  sr_1=lo  arith_type1=Unsigned  bin_pt1=0  sr_2=hi  arith_type2=Unsigned  bin_pt2=0  sr_3=3  arith_type3=Unsigned  bin_pt3=0  sr_4=4  arith_type4=Unsigned  bin_pt4=0  XmcBlockStatus=1  maskContainerNames=group1  block_type=bitbasher  block_config=sysgen:BitBasher_config
      | lo={in[31:0]}
      | hi={in[63:32]}
  BitBasher3 : hdlBasic/BitBasher  bitexpr=|  display_expr=off  sr_1=lo  arith_type1=Unsigned  bin_pt1=0  sr_2=hi  arith_type2=Unsigned  bin_pt2=0  sr_3=3  arith_type3=Unsigned  bin_pt3=0  sr_4=4  arith_type4=Unsigned  bin_pt4=0  XmcBlockStatus=1  maskContainerNames=group1  block_type=bitbasher  block_config=sysgen:BitBasher_config
      | lo={in[31:0]}
      | hi={in[63:32]}
  Delay{,1..7} (8 alike) : hdlBasic/Delay  rst=off  en=off  latency=1  reg_retiming=off  XmcBlockStatus=1  maskContainerNames=group1  block_type=delay  block_config=sysgen:Delay_config
  Logical : hdlBasic/Logical  logical_function=AND  inputs=4  en=off  latency=0  precision=Full  arith_type=Unsigned  n_bits=16  bin_pt=0  align_bp=on  overflow=[]  quantization=[]  XmcBlockStatus=1  maskContainerNames=tabcontainer1  block_type=logical  block_config=sysgen:Logical_config
  Logical1 : hdlBasic/Logical  logical_function=AND  inputs=2  en=off  latency=1  precision=Full  arith_type=Unsigned  n_bits=16  bin_pt=0  align_bp=on  overflow=[]  quantization=[]  XmcBlockStatus=1  maskContainerNames=tabcontainer1  block_type=logical  block_config=sysgen:Logical_config
  P{0..7} (8 alike) : hdlBasic/Gateway Out  inherit_from_input=on  hdl_port=on  rows=1  columns=1  UseAsDAC=off  DACChannel='1'  interface=None  automatic_assignment=on  address_offset=hex2dec('00')  intf_name=''  intf_description=''  timing_constraint=None  locs_specified=off  LOCs={}  io_standard={}  XmcBlockStatus=1  maskContainerNames=group4  block_type=gatewayout  block_config=sysgen:gateway_out_config
  ValidOut : hdlBasic/Gateway Out  inherit_from_input=on  hdl_port=on  rows=1  columns=1  UseAsDAC=off  DACChannel='1'  interface=None  automatic_assignment=on  address_offset=hex2dec('00')  intf_name=''  intf_description=''  timing_constraint=None  locs_specified=off  LOCs={}  io_standard={}  XmcBlockStatus=1  maskContainerNames=group4  block_type=gatewayout  block_config=sysgen:gateway_out_config
  in1_tdata : hdlBasic/Gateway In  gui_display_data_type=Fixed-point  arith_type=Unsigned  n_bits=64  bin_pt=0  preci_type=Single  exp_width=8  frac_width=24  rows=1  columns=1  quantization="Round  (unbiased: +/- Inf)"  overflow=Saturate  period=1  UseAsADC=off  ADCChannel='1'  interface=None  automatic_assignment=on  address_offset=hex2dec('00')  intf_name=''  intf_description=''  default_value=0  timing_constraint=None  locs_specified=off  LOCs={}  io_standard={}  inherit_from_input=off  hdl_port=on  XmcBlockStatus=1  maskContainerNames=group4  block_type=gatewayin  block_config=sysgen:gateway_in_config
  in1_tready : hdlBasic/Gateway Out  inherit_from_input=on  hdl_port=on  rows=1  columns=1  UseAsDAC=off  DACChannel='1'  interface=None  automatic_assignment=on  address_offset=hex2dec('00')  intf_name=''  intf_description=''  timing_constraint=None  locs_specified=off  LOCs={}  io_standard={}  XmcBlockStatus=1  maskContainerNames=group4  block_type=gatewayout  block_config=sysgen:gateway_out_config
  in1_tvalid : hdlBasic/Gateway In  gui_display_data_type=Boolean  arith_type=Boolean  n_bits=16  bin_pt=14  preci_type=Single  exp_width=8  frac_width=24  rows=1  columns=1  quantization="Round  (unbiased: +/- Inf)"  overflow=Saturate  period=1  UseAsADC=off  ADCChannel='1'  interface=None  automatic_assignment=on  address_offset=hex2dec('00')  intf_name=''  intf_description=''  default_value=0  timing_constraint=None  locs_specified=off  LOCs={}  io_standard={}  inherit_from_input=off  hdl_port=on  XmcBlockStatus=1  maskContainerNames=group4  block_type=gatewayin  block_config=sysgen:gateway_in_config
  in2_tdata : hdlBasic/Gateway In  gui_display_data_type=Fixed-point  arith_type=Unsigned  n_bits=64  bin_pt=0  preci_type=Single  exp_width=8  frac_width=24  rows=1  columns=1  quantization="Round  (unbiased: +/- Inf)"  overflow=Saturate  period=1  UseAsADC=off  ADCChannel='1'  interface=None  automatic_assignment=on  address_offset=hex2dec('00')  intf_name=''  intf_description=''  default_value=0  timing_constraint=None  locs_specified=off  LOCs={}  io_standard={}  inherit_from_input=off  hdl_port=on  XmcBlockStatus=1  maskContainerNames=group4  block_type=gatewayin  block_config=sysgen:gateway_in_config
  in2_tready : hdlBasic/Gateway Out  inherit_from_input=on  hdl_port=on  rows=1  columns=1  UseAsDAC=off  DACChannel='1'  interface=None  automatic_assignment=on  address_offset=hex2dec('00')  intf_name=''  intf_description=''  timing_constraint=None  locs_specified=off  LOCs={}  io_standard={}  XmcBlockStatus=1  maskContainerNames=group4  block_type=gatewayout  block_config=sysgen:gateway_out_config
  in2_tvalid : hdlBasic/Gateway In  gui_display_data_type=Boolean  arith_type=Boolean  n_bits=16  bin_pt=14  preci_type=Single  exp_width=8  frac_width=24  rows=1  columns=1  quantization="Round  (unbiased: +/- Inf)"  overflow=Saturate  period=1  UseAsADC=off  ADCChannel='1'  interface=None  automatic_assignment=on  address_offset=hex2dec('00')  intf_name=''  intf_description=''  default_value=0  timing_constraint=None  locs_specified=off  LOCs={}  io_standard={}  inherit_from_input=off  hdl_port=on  XmcBlockStatus=1  maskContainerNames=group4  block_type=gatewayin  block_config=sysgen:gateway_in_config
  in3_tdata : hdlBasic/Gateway In  gui_display_data_type=Fixed-point  arith_type=Unsigned  n_bits=64  bin_pt=0  preci_type=Single  exp_width=8  frac_width=24  rows=1  columns=1  quantization="Round  (unbiased: +/- Inf)"  overflow=Saturate  period=1  UseAsADC=off  ADCChannel='1'  interface=None  automatic_assignment=on  address_offset=hex2dec('00')  intf_name=''  intf_description=''  default_value=0  timing_constraint=None  locs_specified=off  LOCs={}  io_standard={}  inherit_from_input=off  hdl_port=on  XmcBlockStatus=1  maskContainerNames=group4  block_type=gatewayin  block_config=sysgen:gateway_in_config
  in3_tready : hdlBasic/Gateway Out  inherit_from_input=on  hdl_port=on  rows=1  columns=1  UseAsDAC=off  DACChannel='1'  interface=None  automatic_assignment=on  address_offset=hex2dec('00')  intf_name=''  intf_description=''  timing_constraint=None  locs_specified=off  LOCs={}  io_standard={}  XmcBlockStatus=1  maskContainerNames=group4  block_type=gatewayout  block_config=sysgen:gateway_out_config
  in3_tvalid : hdlBasic/Gateway In  gui_display_data_type=Boolean  arith_type=Boolean  n_bits=16  bin_pt=14  preci_type=Single  exp_width=8  frac_width=24  rows=1  columns=1  quantization="Round  (unbiased: +/- Inf)"  overflow=Saturate  period=1  UseAsADC=off  ADCChannel='1'  interface=None  automatic_assignment=on  address_offset=hex2dec('00')  intf_name=''  intf_description=''  default_value=0  timing_constraint=None  locs_specified=off  LOCs={}  io_standard={}  inherit_from_input=off  hdl_port=on  XmcBlockStatus=1  maskContainerNames=group4  block_type=gatewayin  block_config=sysgen:gateway_in_config
  in4_tdata : hdlBasic/Gateway In  gui_display_data_type=Fixed-point  arith_type=Unsigned  n_bits=64  bin_pt=0  preci_type=Single  exp_width=8  frac_width=24  rows=1  columns=1  quantization="Round  (unbiased: +/- Inf)"  overflow=Saturate  period=1  UseAsADC=off  ADCChannel='1'  interface=None  automatic_assignment=on  address_offset=hex2dec('00')  intf_name=''  intf_description=''  default_value=0  timing_constraint=None  locs_specified=off  LOCs={}  io_standard={}  inherit_from_input=off  hdl_port=on  XmcBlockStatus=1  maskContainerNames=group4  block_type=gatewayin  block_config=sysgen:gateway_in_config
  in4_tready : hdlBasic/Gateway Out  inherit_from_input=on  hdl_port=on  rows=1  columns=1  UseAsDAC=off  DACChannel='1'  interface=None  automatic_assignment=on  address_offset=hex2dec('00')  intf_name=''  intf_description=''  timing_constraint=None  locs_specified=off  LOCs={}  io_standard={}  XmcBlockStatus=1  maskContainerNames=group4  block_type=gatewayout  block_config=sysgen:gateway_out_config
  in4_tvalid : hdlBasic/Gateway In  gui_display_data_type=Boolean  arith_type=Boolean  n_bits=16  bin_pt=14  preci_type=Single  exp_width=8  frac_width=24  rows=1  columns=1  quantization="Round  (unbiased: +/- Inf)"  overflow=Saturate  period=1  UseAsADC=off  ADCChannel='1'  interface=None  automatic_assignment=on  address_offset=hex2dec('00')  intf_name=''  intf_description=''  default_value=0  timing_constraint=None  locs_specified=off  LOCs={}  io_standard={}  inherit_from_input=off  hdl_port=on  XmcBlockStatus=1  maskContainerNames=group4  block_type=gatewayin  block_config=sysgen:gateway_in_config
  Out2 : Outport
  Out3 : Outport  Port=2
  Out4 : Outport  Port=3
  Out5 : Outport  Port=4
  Out7 : Outport  Port=5
  Out8 : Outport  Port=6
  Out9 : Outport  Port=7
  Out11 : Outport  Port=8
  Out10 : Outport  Port=9
  Out1 : Outport  Port=10
  Out6 : Outport  Port=11
  Out12 : Outport  Port=12
  Out13 : Outport  Port=13
  wires:
  BitBasher/1 -> Delay1/1
  Delay2/1 -> P1/1
  AXI FIFO3/3 -> in4_tready/1
  Logical1/1 -> ValidOut/1
  AXI FIFO3/1 -> [Valid3]
  AXI FIFO/2 -> BitBasher/1
  AXI FIFO3/2 -> BitBasher3/1
  AXI FIFO2/3 -> in3_tready/1
  AXI FIFO1/3 -> in2_tready/1
  [Valid2] -> Logical/3
  Delay3/1 -> P5/1
  AXI FIFO1/1 -> [Valid1]
  BitBasher3/1 -> Delay7/1
  in4_tvalid/1 -> AXI FIFO3/2
  ValidOut/1 -> Out10/1
  P4/1 -> Out7/1
  P5/1 -> Out8/1
  P3/1 -> Out5/1
  in4_tdata/1 -> AXI FIFO3/3
  BitBasher2/2 -> Delay4/1
  P0/1 -> Out2/1
  in3_tready/1 -> Out12/1
  in1_tvalid/1 -> AXI FIFO/2
  In7/1 -> in4_tdata/1
  P2/1 -> Out4/1
  BitBasher1/2 -> Delay3/1
  AXI FIFO/1 -> Logical1/2, [Valid0]
  In2/1 -> in1_tvalid/1
  Delay1/1 -> P0/1
  P6/1 -> Out9/1
  in2_tready/1 -> Out6/1
  in3_tdata/1 -> AXI FIFO2/3
  BitBasher/2 -> Delay/1
  [Valid0] -> Logical/1
  In4/1 -> in2_tvalid/1
  In6/1 -> in3_tvalid/1
  BitBasher1/1 -> Delay2/1
  in3_tvalid/1 -> AXI FIFO2/2
  in1_tready/1 -> Out1/1
  in1_tdata/1 -> AXI FIFO/3
  P1/1 -> Out3/1
  In3/1 -> in2_tdata/1
  in4_tready/1 -> Out13/1
  AXI FIFO2/2 -> BitBasher2/1
  Delay/1 -> P4/1
  In1/1 -> in1_tdata/1
  P7/1 -> Out11/1
  [Valid3] -> Logical/4
  Delay7/1 -> P3/1
  in2_tvalid/1 -> AXI FIFO1/2
  Delay5/1 -> P7/1
  Delay4/1 -> P6/1
  in2_tdata/1 -> AXI FIFO1/3
  [Valid1] -> Logical/2
  In8/1 -> in4_tvalid/1
  AXI FIFO2/1 -> [Valid2]
  AXI FIFO/3 -> in1_tready/1
  In5/1 -> in3_tdata/1
  AXI FIFO1/2 -> BitBasher1/1
  BitBasher3/2 -> Delay5/1
  BitBasher2/1 -> Delay6/1
  Delay6/1 -> P2/1
  Logical/1 -> Logical1/1, AXI FIFO/1, AXI FIFO1/1, AXI FIFO2/1, AXI FIFO3/1
